simulink model "simulink_mode"  (R2023b)
settings: Solver=ode4  StartTime=0.0  StopTime=20  FixedStep=0.01  RelTol=1e-3
model workspace (MATLAB code in the model file):
  | m               = 12;                       % Mass in kg
  | Ixx             = 1.86;                     % Ixx in kgm^2
  | Iyy             = 2.031;                    % Iyy in kgm^2
  | Ixy             = 0;                        % Ixy in kgm^2
  | Ixz             = 0;                        % Ixz in kgm^2
  | Iyz             = 0;                        % Iyz in kgm^2
  | Izz             = 3.617;                    % Izz in kgm^2
  | g               = 9.81;
  | b               = 0.032;                        % Blade chord in m
  | l               = 0.40;                         % Arm length in m
  | RPM             = 3000;
  | omega_w         = 2 * pi * RPM / 60;            % Ang vel in rad/s
  | R               = 0.355;                        % Blade radius in meters
  | rho             = 1.225;                        % Air density in kg/m^3
  | K               = rho * pi * R^2 * (omega_w * R)^2;   % Constant K
  | V_tip           = omega_w * R;                        % Blade tip velocity in m/s
  | blade_area      = pi * R^2;                     % Blade area
  | CT_init         = (0.25*m*g/(rho*blade_area*V_tip^2));
  | I = diag([Ixx, Iyy, Izz]);
  | 
  | %% Gains
  | zeta_quat = diag([0.95, 0.95, 0.95, 0.95]);
  | omega_n_quat = diag([25, 25, 25, 25]);
  | 
  | zeta_x = diag([0.95, 0.95, 0.95]);
  |     omega_n_x = diag([10, 10, 15]);
settings Model: Creator=dsai9  LastModifiedBy=dsai9

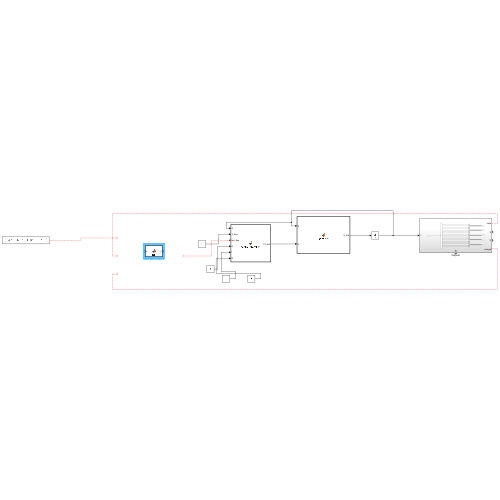
[thumbnail: Simulink's stored preview of the top-level diagram]
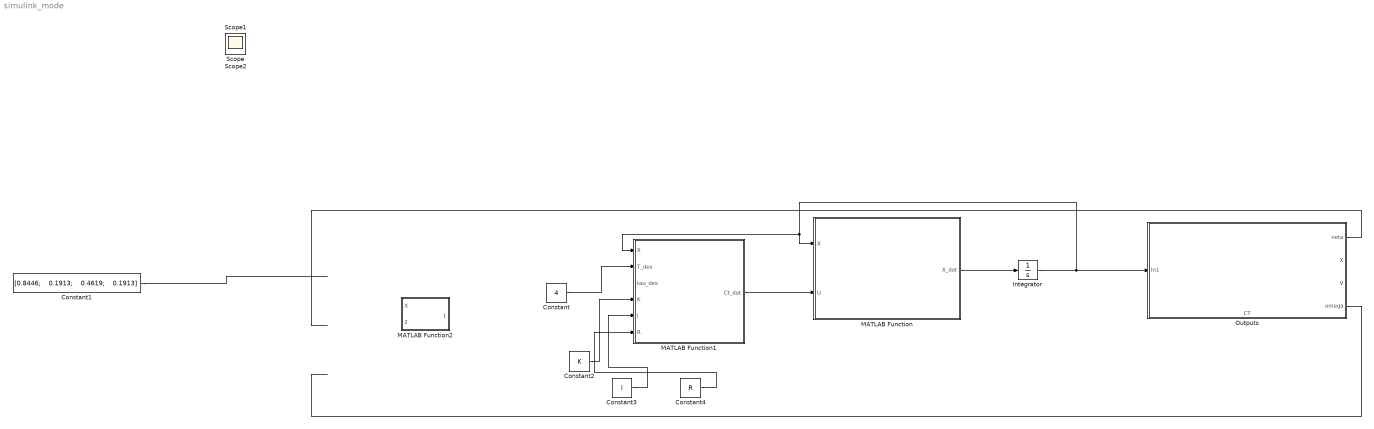
== system simulink_mode ==
  Constant : Constant  Value=4
  Constant1 : Constant  Value="[0.8446;    0.1913;    0.4619;    0.1913]"
  Constant2 : Constant  Value=K
  Constant3 : Constant  Value=l
  Constant4 : Constant  Value=R
  Integrator : Integrator  InitialCondition=[0; 0; 0; 0; 0; 0; 1; 0; 0; 0; 0; 0; 0; 0.004; 0.004; 0.004; 0.004];
  MATLAB Function : MATLAB Function  TreatAsAtomicUnit=on
  MATLAB Function1 : MATLAB Function  TreatAsAtomicUnit=on
  MATLAB Function2 : MATLAB Function  TreatAsAtomicUnit=on
  Outputs : Subsystem
      settings: PortSchema="{\"entries\":[{\"content\":{\"sides\":[{\"content\":{\"connectorIds\":[\"In1\"]},\"type\":\"ConnectorPlacement.EquallySpacedRectSide\",\"uuid\":\"dfed46bb-4077-4d2c-a6e0-595fd02d135c\"},{\"content\":{\"connectorIds\":[\"Out1\",\"Out2\",\"Out3\",\"Out4\"],\"side\":\"RIGHT\"},\"type\":\"ConnectorPlacement.EquallySpacedRectSide\",\"uuid\":\"89f2e8ce-3964-4221-b3a8-6a078739bdb5\"},{\"content\":{\"side\":\"TOP\"},\"type\":\"ConnectorPlacement.EquallySpacedRectSide\",\"uuid\":\"cbab99cd-c426-42c4-87c8-a5dedb5e7b77\"},{\"content\":{\"connectorIds\":[\"Out5\"],\"side\":\"BOTTOM\"},\"type\":\"ConnectorPlacement.EquallySpacedRectSide\",\"uuid\":\"c7bf5d86-9e42-4b85-bdd0-649fd8831b9f\"}]},\"type\":\"ConnectorPlacement.EquallySpacedConnector\",\"uuid\":\"d1cf55fe-096b-4063-b50c-4176128d5459\"}],\"packageUris\":[\"http://schema.mathworks.com/mf0/Connector/R2020b\"],\"version\":\"1.0\"}"
  Scope : Scope
  Scope1 : Scope
  Scope2 : Scope
  wires:
  MATLAB Function/1(X_dot) -> Integrator/1
  Integrator/1 -> Outputs/1(In1), MATLAB Function/1(X), MATLAB Function1/1(X)
  MATLAB Function1/1(Ct_dot) -> MATLAB Function/2(U)
  Constant/1 -> MATLAB Function1/2(T_des)
  ? -> MATLAB Function1/3(tau_des)
  Constant1/1 -> ?
  Outputs/1(neta) -> ?
  Outputs/4(omega) -> ?
  Constant2/1 -> MATLAB Function1/4(K)
  Constant3/1 -> MATLAB Function1/5(l)
  Constant4/1 -> MATLAB Function1/6(R)

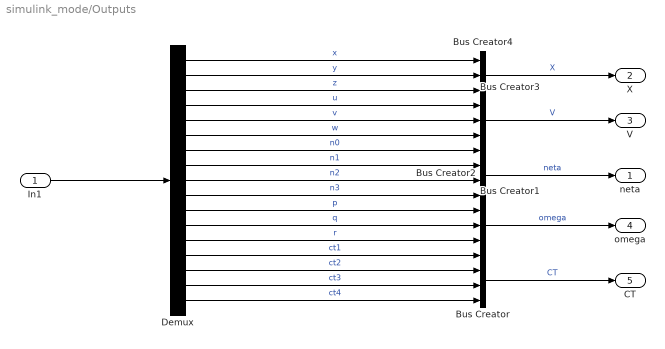
== system simulink_mode/Outputs ==
  In1 : Inport
  Bus Creator : BusCreator  Inputs=4
  Bus Creator1 : BusCreator  Inputs=3
  Bus Creator2 : BusCreator  Inputs=4
  Bus Creator3 : BusCreator  Inputs=3
  Bus Creator4 : BusCreator  Inputs=3
  Demux : Demux  Outputs=17
  neta : Outport
  X : Outport  Port=2
  V : Outport  Port=3
  omega : Outport  Port=4
  CT : Outport  Port=5
  wires:
  Demux/6 -> Bus Creator3/3  "w"
  Demux/3 -> Bus Creator4/3  "z"
  Demux/7 -> Bus Creator2/1  "n0"
  Bus Creator4/1 -> X/1  "X"
  Demux/16 -> Bus Creator/3  "ct3"
  Demux/17 -> Bus Creator/4  "ct4"
  Demux/10 -> Bus Creator2/4  "n3"
  Demux/14 -> Bus Creator/1  "ct1"
  Demux/15 -> Bus Creator/2  "ct2"
  Demux/13 -> Bus Creator1/3  "r"
  Demux/11 -> Bus Creator1/1  "p"
  Demux/2 -> Bus Creator4/2  "y"
  Demux/12 -> Bus Creator1/2  "q"
  Demux/9 -> Bus Creator2/3  "n2"
  Demux/8 -> Bus Creator2/2  "n1"
  Demux/5 -> Bus Creator3/2  "v"
  Demux/4 -> Bus Creator3/1  "u"
  Demux/1 -> Bus Creator4/1  "x"
  Bus Creator1/1 -> omega/1  "omega"
  Bus Creator/1 -> CT/1  "CT"
  Bus Creator3/1 -> V/1  "V"
  In1/1 -> Demux/1
  Bus Creator2/1 -> neta/1  "neta"

== matlab function simulink_mode/MATLAB Function1 ==
  data: X input; Ct_dot output; T_des input; tau_des input; K input; l input; R input
function Ct_dot  = control_allocation(X, T_des, tau_des, K, l, R)
    


ct1 = X(14);
ct2 = X(15);
ct3 = X(16);
ct4 = X(17);

kt = 125;
kl = 125;
km = 125;
kn = 1000;
T = K*(ct1 + ct2 + ct3 + ct4);
L_tbar = K * l *(ct1 - ct2 - ct3 + ct4);
M_t = K * l * (ct1 + ct2 - ct3 - ct4);
N_t = (K*R/sqrt(2)) * (abs(ct1)^1.5 - abs(ct2)^1.5 + abs(ct3)^1.5 - abs(ct4)^1.5);

L_t_bar_des = tau_des(1);
M_t_des = tau_des(2);
N_t_des = tau_des(3);

thrust_tau_dot_err = [kt*(T_des - T);
                      kl*(L_t_bar_des - L_tbar);
                      km*(M_t_des - M_t);
                      kn*(N_t_des - N_t)];
mixing_matrix = [K K K K;
                 K*l -K*l -K*l K*l;
                 K*l K*l -K*l -K*l;
                 (3*K*R/2)*sqrt(abs(ct1)/2) -(3*K*R/2)*sqrt(abs(ct2)/2) (3*K*R/2)*sqrt(abs(ct3)/2) -(3*K*R/2)*sqrt(abs(ct4)/2)];
Ct_dot = pinv(mixing_matrix)*thrust_tau_dot_err;

end

== matlab function simulink_mode/MATLAB Function ==
  settings: updateMethod=DISCRETE  sampleTime=0.01
  data: X input double size=[17,1]; X_dot output double size=[17,1]; U input double size=[4,1]
function X_dot = dynamics2(X,U)

% k_t = 1e-3; % Thrust Coefficient

%% Parameters
m               = 12;                       % Mass in kg
g               = 9.81;   
l               = 0.40;                         % Arm length in m
rho = 1.225;
R               = 0.355;   
omega_w = 3000;
K               = rho * pi * R^2 * (omega_w * R)^2;



I = diag([1.86, 2.031, 3.617]);
I_x = I(1,1);
I_y = I(2,2);
I_z = I(3,3);
I_xz = 0;


%% State Unpacking
% w1 = u(1);
% w2 = u(2);
% w3 = u(3);
% w4 = u(4);



% Linear Velocity
u = X(4);
v = X(5);
w = X(6);

% Orientation In Quaternion
n0 = X(7);
n1 = X(8);
n2 = X(9);
n3 = X(10);

% Angular Velocity
p = X(11);
q = X(12);
r = X(13);

% Thrust Coefficients
ct1 = X(14);
ct2 = X(15);
ct3 = X(16);
ct4 = X(17);

%% Aero Dynamic Forces (TBD)
F_ax = 0;
F_ay = 0;
F_az = 0;

L_abar = 0;
% L_tbar = 0;
M_a = 0;
% M_t = 0;
N_a = 0;
% N_t = 0;


%% Constants
C1 = (1/(I_x*I_z - I_xz)) .* [(I_y - I_z)*I_z - I_xz^2;
                             (I_x - I_y + I_z)*I_xz;
                             I_z;
                             I_xz;
                             (I_x - I_y)*I_x + I_xz^2;
                             I_x];
c1 = C1(1);
c2 = C1(2);
c3 = C1(3);
c4 = C1(4);
c8 = C1(5);
c9 = C1(6);

C2 = (1/I_y) .*  [(I_z - I_x);
                  I_xz;
                  1];

c5 = C2(1);
c6 = C2(2);
c7 = C2(3);

%% Control Allocation
T = K*(ct1 + ct2 + ct3 + ct4);
L_tbar = K * l *(ct1 - ct2 - ct3 + ct4);
M_t = K * l * (ct1 + ct2 - ct3 - ct4);
N_t = (K*R/sqrt(2)) * (abs(ct1)^1.5 - abs(ct2)^1.5 + abs(ct3)^1.5 - abs(ct4)^1.5);
%% True Air Speed and Dynamic Pressure
% rho = 1.225;
% V = sqrt(u^2 + v^2 + w^2);
% Q_inf = 0.5*rho*V^2;


% Rotation Matrices
Rot_mat_body2iner_inquat = [n0^2+n1^2-n2^2-n3^2, (2*n1*n2)-(2*n3*n0), (2*n1*n3) + (2*n2*n0);
                     (2*n1*n2)+(2*n3*n0), (n0^2-n1^2+n2^2-n3^2), (2*n2*n3)-(2*n0*n1);
                     (2*n1*n3)-(2*n2*n0), (2*n2*n3+2*n1*n0), (n0^2-n1^2-n2^2+n3^2)];

%% Dynamics
% T = k_t*(w1^2 + w2^2 + w3^2 + w4^2);
lin_vel_dot = [0; 0; -T/m] + [F_ax/m; F_ay/m; F_az/m] +g .* [2*n1*n3 - 2*n0*n2; 2*n2*n3 + 2*n0*n1; n0^2-n1^2-n2^2+n3^2] + [r*v - q*w; p*w - r*u; q*u - p*v];
ang_vel_dot = [(c1*r + c2*p)*q + c3*(L_abar + L_tbar) + c4*(N_a + N_t);
                c5*p*r - c6*(p^2 - r^2) + c7*(M_a + M_t);
                (c8*p - c2*r)*q + c4*(L_abar + L_tbar) + c9*(N_a + N_t)];

%% Kinematics 
pos_dot = Rot_mat_body2iner_inquat*[u; v; w];
n_dot = 0.5 .* [-n1, -n2, -n3;
                n0, -n3, n2;
                n3, n0, -n1;
                -n2, n1, n0] * [p; q; r];

%% Inputs
ct_dot = U;

X_dot = [pos_dot; lin_vel_dot; n_dot; ang_vel_dot; ct_dot];

== matlab function simulink_mode/MATLAB Function2 ==
  data: X input; Moments_t_des output; neta_des input
function Moments_t_des = inner_loop(X, neta_des)

% X(4:7) = Quaternions
% Quater_d        = Xd(7:11);
neta_d = neta_des';
neta         = X(7:10)';
omega      = X(11:13)';

parameters;

neta_d = neta_d / norm(neta_d);

neta_d_conj = quaternConj(neta_d);


neta_e = quaternProd(neta_d_conj', neta);

neta_e = neta_e / norm(neta_e);


a1 = quaternProd(neta_e, [0, omega]);



omega_d = quaternProd(a1, quaternConj(neta_e));


omega_e = omega' - quat2rotm(neta_e)' * omega_d(2:4)';


neta_e_dot = 0.5*quaternProd(neta_e, [0;omega_e]);

neta_err_dot = 0.5 * quaternProd([-neta_e(2:4), neta_e(1)], neta_e_dot);






neta_err_des = [1; 0; 0; 0];



neta_err_ddot = -(2 * zeta_quat * omega_n_quat' * neta_err_dot') - (omega_n_quat * omega_n_quat' * (neta_e' - neta_err_des));



G = calculate_G(neta_e);

omega_e_dot = 2*G*neta_err_ddot;


Moments_t_des = I*omega_e_dot + cross(omega', I*omega');

neta_err_ddot

end
